simulink model "thrusttoVel"  (R2026a)
settings: Solver=FixedStepDiscrete  StopTime=60  FixedStep=0.01
undefined symbols (not defined in the file or in its folder): DiscIntNeverNeededParam
settings Model: Creator=husey  LastModifiedBy=husey
settings DebuggingCC: InheritedTsInSrcMsg=none

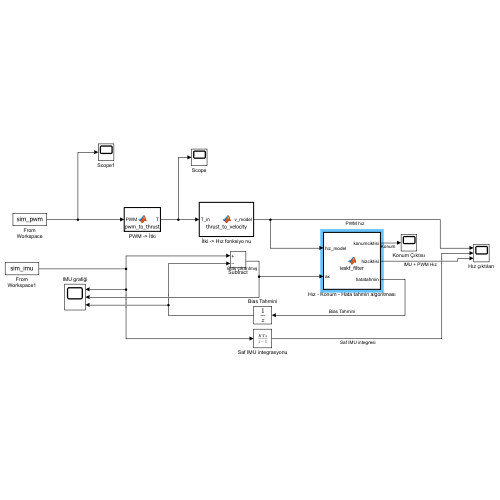
[thumbnail: Simulink's stored preview of the top-level diagram]
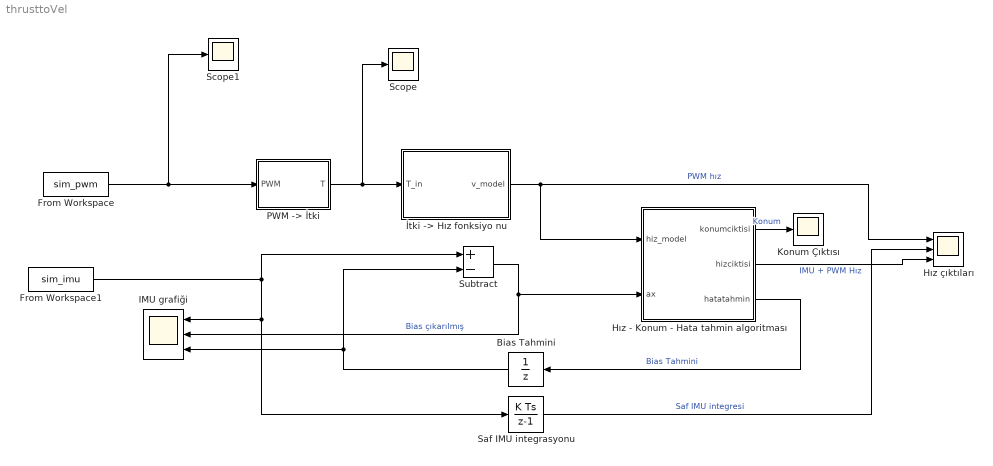
== system thrusttoVel ==
  Bias Tahmini : UnitDelay  SampleTime=-1
  From Workspace : FromWorkspace  VariableName=sim_pwm
  From Workspace1 : FromWorkspace  VariableName=sim_imu  OutDataTypeStr=double  SampleTime=-1  OutputAfterFinalValue=Setting to zero
  Hız - Konum - Hata tahmin algoritması : MATLAB Function  TreatAsAtomicUnit=on
  Hız çıktıları : Scope  NumInputPorts=3
      settings: ActiveDisplayYMinimum=-0.95127068737277121  ActiveDisplayYMaximum=2.0609519165039774
  IMU grafiği : Scope  NumInputPorts=3
      settings: ActiveDisplayYMinimum=-36502.661409736393  ActiveDisplayYMaximum=46142.827776574355
  Konum Çıktısı : Scope
      settings: ActiveDisplayYMinimum=8.5247703386239859  ActiveDisplayYMaximum=11.1471518834207
  "PWM -> İtki" : MATLAB Function  TreatAsAtomicUnit=on
  Saf IMU integrasyonu : DiscreteIntegrator  SampleTime=-1  ICPrevOutput=DiscIntNeverNeededParam  ICPrevScaledInput=DiscIntNeverNeededParam
  Scope : Scope
      settings: ActiveDisplayYMinimum=-60.119378396656913  ActiveDisplayYMaximum=42.702402740587132
  Scope1 : Scope
      settings: ActiveDisplayYMinimum=632.8191011686622  ActiveDisplayYMaximum=1635.5771152066152  DataLoggingVariableName=ScopeData2
  Subtract : Sum  Inputs=+-
  "İtki -> Hız fonksiyo nu" : MATLAB Function  TreatAsAtomicUnit=on
  wires:
  From Workspace/1 -> Scope1/1, "PWM -> İtki"/1(PWM)
  "PWM -> İtki"/1(T) -> Scope/1, "İtki -> Hız fonksiyo nu"/1(T_in)
  "İtki -> Hız fonksiyo nu"/1(v_model) -> Hız çıktıları/1, Hız - Konum - Hata tahmin algoritması/1(hiz_model)  "PWM hız"
  Subtract/1 -> IMU grafiği/2, Hız - Konum - Hata tahmin algoritması/2(ax)  "Bias çıkarılmış"
  Hız - Konum - Hata tahmin algoritması/2(hizciktisi) -> Hız çıktıları/3  "IMU + PWM Hız"
  Hız - Konum - Hata tahmin algoritması/3(hatatahmin) -> Bias Tahmini/1  "Bias Tahmini"
  Bias Tahmini/1 -> IMU grafiği/3, Subtract/2
  From Workspace1/1 -> Subtract/1, Saf IMU integrasyonu/1, IMU grafiği/1
  Saf IMU integrasyonu/1 -> Hız çıktıları/2  "Saf IMU integresi"
  Hız - Konum - Hata tahmin algoritması/1(konumciktisi) -> Konum Çıktısı/1  "Konum"

== matlab function thrusttoVel/Hız - Konum - Hata tahmin algoritması ==
  data: konumciktisi output; hiz_model input; hizciktisi output; ax input; hatatahmin output
function [konumciktisi, hizciktisi, hatatahmin] = ieskf_filter(hiz_model, ax)
    persistent P v_est bias_est x_est hiz_model_eski initialized counter zupt_counter
    
    dt_predict = 0.01; 
    
    if isempty(initialized)
        P = [0.01, 0;  
             0,    0.01]; 
        v_est = 0;     
        bias_est = 0;
        x_est = 0;   
        hiz_model_eski = 0; 
        counter = 0; 
        zupt_counter = 0;
        initialized = true;
    end
    
    % ==========================================
    % 1. KONUM ENTEGRASYONU 
    % ==========================================
    x_est = x_est + ((hiz_model_eski + hiz_model) / 2) * dt_predict; 
    hiz_model_eski = hiz_model;
    
    % ==========================================
    % 2. PREDICT ADIMI (100 Hz)
    % ==========================================
    ivme_temiz = ax - bias_est; 
    
    v_est = v_est + ivme_temiz * dt_predict;
    
    F = [1, -dt_predict;
         0,  1 ];
         
    Q = [0.01,  0;    
         0,     1e-4]; 
         
    P = F * P * F' + Q;
    
    % ==========================================
    % 3. UPDATE ADIMI
    % ==========================================
    counter = counter + 1;
    
    if counter >= 2 
        R = 1e-4; 
        
        H = [1, 0]; 
        x_err = [0; 0];
        max_iter = 3;
        
        for i = 1:max_iter
            z = hiz_model - (v_est + x_err(1)); 
            
            S = H * P * H' + R;
            K = (P * H') / S;
            
            x_err = x_err + K * z;
            
            if abs(z) < 1e-4
                break;
            end
        end
        
        P = (eye(2) - K * H) * P;
        
        v_est = v_est + x_err(1);
        bias_est = bias_est + x_err(2);
        
        counter = 0; 
    end
    
    % ==========================================
    % 4. GÜVENLİ ZUPT (DURAĞANLIK) KONTROLÜ
    % ==========================================
    % Rastgele gürültülerin veya sabit hızlı seyirlerin yanlışlıkla ZUPT tetiklemesini 
    % önlemek için koşulların ARKA ARKAYA birkaç döngü boyunca sağlanması gerekir.
    
    is_model_zero = (hiz_model == 0);
    is_acc_quiet  = (abs(ivme_temiz) < 0.04);
    
    if is_model_zero && is_acc_quiet
        zupt_counter = zupt_counter + 1;
    else
        zupt_counter = 0; % Koşul bozulursa sayacı sıfırla (gürültü filtresi)
    end
    
    % Eğer araç gerçekten 50 adım boyunca (0.5 saniye) hem ıssız hem motorsuz kaldıysa durmuştur
    if zupt_counter >= 50 
        v_est = 0; 
        zupt_counter = 50; % Sayaç taşmasını önle
    end

    % --- ÇIKIŞLAR ---
    konumciktisi = x_est;   
    hizciktisi = v_est;        
    hatatahmin = bias_est; 
end

== matlab function thrusttoVel/İtki -> Hız fonksiyo nu ==
  data: T_in input; v_model output
function v_model = thrust_to_velocity(T_in)
    dt = 0.01; 
    
    persistent v_model_pred initialized
    if isempty(initialized)
        v_model_pred = 0; 
        initialized = true;
    end
    
    % --- 1. MATEMATİKSEL İTKİ KALİBRASYONU ---
    % 50m -> 40.5m dönüşümü için itki çarpanı tam 0.65'e (K_thrust) sabitlendi.
    % Bu, aracın gerçek dünyadaki hidrodinamik itki verimidir.
    K_thrust = 0.65; 
    T = T_in * K_thrust; 
    
    % --- 2. SABİT FİZİKSEL PARAMETRELER ---
    rho = 1000;  
    A = 0.0176; 
    m = 11.209 * 1.05; 
    Cd_cfd = 0.22; % Saf gövde sürtünmesi
    
    % --- 3. SÜRTÜNME HESAPLAMALARI ---
    Fd_hull = 0.5 * rho * Cd_cfd * A * (v_model_pred^2) * sign(v_model_pred);
    
    % Lineer sürtünme dengede bırakıldı (aşırı frenlememesi için)
    Cd_lin = 0.15; 
    Fd_lin = Cd_lin * v_model_pred;
    
    Fd_prop = 0;
    if T <= 0
        Cp_prop = 0.02; 
        Fd_prop = 0.5 * rho * Cp_prop * A * (v_model_pred^2) * sign(v_model_pred);
    end
    
    Fd_total = Fd_hull + Fd_lin + Fd_prop;
    
    % İvme hesabı 
    a_model = (T - Fd_total) / m;
    v_model_pred = v_model_pred + a_model * dt;
  
    if T <= 0 && abs(v_model_pred) < 0.02
        v_model_pred = 0;
    end
    
    v_model = v_model_pred;
end

== matlab function thrusttoVel/PWM -> İtki ==
  data: PWM input; T output
function T = pwm_to_thrust(PWM)
    % 1. Sinyal Sınırlandırma
    if PWM < 1000
        PWM = 1000;
    elseif PWM > 2000
        PWM = 2000;
    end
    
    % 2. Ölü Bölge Kontrolü
    if PWM < 1050
        T = 0.0;
    else
        % --- 4S VE 24V GRAFİK GERÇEĞİNE GÖRE İTKİ HESABI ---
        % Eski harmanlanmış karmaşık yapı yerine, datasheet grafiğindeki 
        % pürüzsüz karesel eğriyi (parabol) ve 4S voltaj düşümünü kullanıyoruz.
        
        % (14.8V / 24.0V)^2 voltaj çarpanı
        VOLTAGE_SCALE_4S = 0.38; 
        
        % Grafikteki 24V max itki (~8.8 kg -> 88 N)
        max_thrust_24v_N = 88.0; 
        
        % 0.0 ile 1.0 arasında normalize edilmiş gaz (Throttle)
        throttle = (PWM - 1000) / 1000;
        
        % Grafikteki 24V itki karakteristiği (Thrust ~ Throttle^2)
        thrust_24v = max_thrust_24v_N * (throttle ^ 2);
        
        % 4S pilin üretebileceği gerçek itki (T)
        T = thrust_24v * VOLTAGE_SCALE_4S;
    end
end
